simulink model "Example_UNO_Traffic_light_task"  (Simulink 3.00)
settings: Solver=ode45  SolverMode=SingleTasking  StartTime=0.0  StopTime=10.0  RelTol=1e-3
libraries: logiclib x40, mathlib x18, genlib x6, speclib x1, execlib x1
settings Model: Creator=Jarda  LastModifiedBy=XPMUser

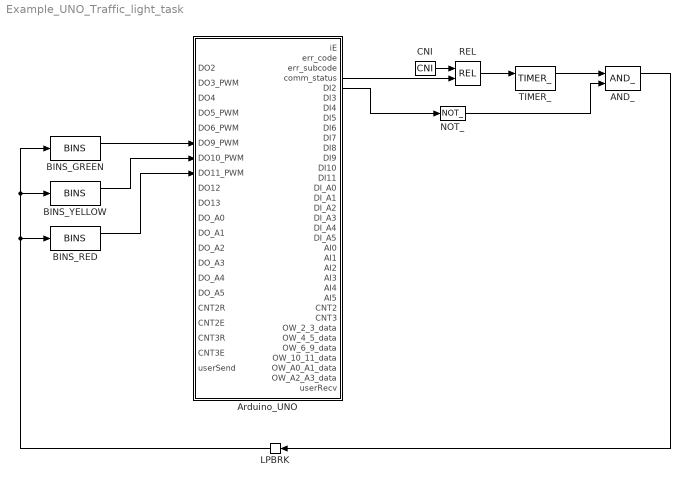
== system Example_UNO_Traffic_light_task ==
  AND_ : logiclib/AND_
  Arduino_UNO : Subsystem  mask(REX sequence){comPort=10, pinmode2=4: Digital input with internal pull-up, pinmode3=1: Not connected, pinmode4=1: Not connected, pinmode5=1: Not connected, pinmode6=1: Not connected, pinmode9=2: Digital output, pinmode10=2: Digital output, pinmode11=2: Digital output, pinmodeA0=1: Not connected, pinmodeA1=1: Not connected, pinmodeA2=1: Not connected, pinmodeA3=1: Not connected, pinmodeA4=1: Not connected, pinmodeA5=1: Not connected}
      mask prompts: comPort "COM port number"; pinmode2 "Pin 2 mode"; pinmode3 "Pin 3 mode"; pinmode4 "Pin 4 mode"; pinmode5 "Pin 5 mode"; pinmode6 "Pin 6 mode"; pinmode9 "Pin 9 mode"; pinmode10 "Pin 10 mode"; pinmode11 "Pin 11 mode"; pinmodeA0 "Analog pin A0 mode"; pinmodeA1 "Analog pin A1 mode"; pinmodeA2 "Analog pin A2 mode"; pinmodeA3 "Analog pin A3 mode"; pinmodeA4 "Analog pin A4 mode"; pinmodeA5 "Analog pin A5 mode"
      mask StyleString: popup(1|2|3|4|5|6|7|8|9|10|11|12),popup(1: Not connected|2: Digital output|3: Digital input|4: Digital input with internal pull-up|5: --- N/A for this pin ---|6: --- N/A for this pin ---|7: 1-Wire temperature|8: Counter|9: Encoder A),popup(1: Not connected|2: Digital output|3: Digital input|4: Digital input with internal pull-up|5: PWM (analog output)|6: --- N/A for this pin ---|7: 1-Wire temperature|8: Counter|9: Encoder A),popup(1: Not connected|2: Digital output|3: Digital input|4: Digital input with internal pull-up|5: --- N/A for this pin ---|6: --- N/A for this pin ---|7: 1-Wire temperature|8: --- N/A for this pin ---|9: --- N/A for this pin ---|10: Counter DIR / Encoder B),popup(1: Not connected|2: Digital output|3: Digital input|4: Digital input with internal pull-up|5: PWM (analog output)|6: --- N/A for this pin ---|7: 1-Wire temperature|8: --- N/A for this pin ---|9: --- N/A for this pin ---|10: Counter DIR / Encoder B),popup(1: Not connected|2: Digital output|3: Digital input|4: Digital input with internal pull-up|5: PWM (analog output)|6: --- N/A for this pin ---|7: 1-Wire temperature),popup(1: Not connected|2: Digital output|3: Digital input|4: Digital input with internal pull-up|5: PWM (analog output)|6: --- N/A for this pin ---|7: 1-Wire temperature),popup(1: Not connected|2: Digital output|3: Digital input|4: Digital input with internal pull-up|5: PWM (analog output)|6: --- N/A for this pin ---|7: 1-Wire temperature),popup(1: Not connected|2: Digital output|3: Digital input|4: Digital input with internal pull-up|5: PWM (analog output)|6: --- N/A for this pin ---|7: 1-Wire temperature),popup(1: Not connected|2: Digital output|3: Digital input|4: Digital input with internal pull-up|5: --- N/A for this pin ---|6: Analog input|7: 1-Wire temperature),popup(1: Not connected|2: Digital output|3: Digital input|4: Digital input with internal pull-up|5: --- N/A for this pin ---|6: Analog input|7: 1-Wire temperature),popup(1: Not connected|2: Digital output|3: Digital input|4: Digital input with internal pull-up|5: --- N/A for this pin ---|6: Analog input|7: 1-Wire temperature),popup(1: Not connected|2: Digital output|3: Digital input|4: Digital input with internal pull-up|5: --- N/A for this pin ---|6: Analog input|7: 1-Wire temperature),popup(1: Not connected|2: Digital output|3: Digital input|4: Digital input with internal pull-up|5: --- N/A for this pin ---|6: Analog input|7: 1-Wire temperature),popup(1: Not connected|2: Digital output|3: Digital input|4: Digital input with internal pull-up|5: --- N/A for this pin ---|6: Analog input|7: 1-Wire temperature)
  BINS_GREEN : genlib/BINS  Y0=on  t1=0  t2=10  t3=0  t4=4  t5=5  t6=6  t7=7  t8=8  RPT=off
  BINS_RED : genlib/BINS  Y0=off  t1=2  t2=10  t3=0  t4=4  t5=5  t6=6  t7=7  t8=8  RPT=off
  BINS_YELLOW : genlib/BINS  Y0=off  t1=0  t2=2  t3=8  t4=10  t5=0  t6=6  t7=7  t8=8  RPT=off
  CNI : mathlib/CNI  icn=3
  LPBRK : execlib/LPBRK  Orientation=left
  NOT_ : logiclib/NOT_
  REL : mathlib/REL  irel=1: equality (==)
  TIMER_ : logiclib/TIMER_  mode=2: Delayed ON  pt=1
  wires:
  AND_/1 -> LPBRK/1
  Arduino_UNO/4(comm_status) -> REL/2
  Arduino_UNO/5(DI2) -> NOT_/1
  BINS_GREEN/1 -> Arduino_UNO/6(DO9_PWM)
  BINS_RED/1 -> Arduino_UNO/8(DO11_PWM)
  BINS_YELLOW/1 -> Arduino_UNO/7(DO10_PWM)
  CNI/1 -> REL/1
  LPBRK/1 -> BINS_RED/1, BINS_GREEN/1, BINS_YELLOW/1
  NOT_/1 -> AND_/2
  REL/1 -> TIMER_/1
  TIMER_/1 -> AND_/1

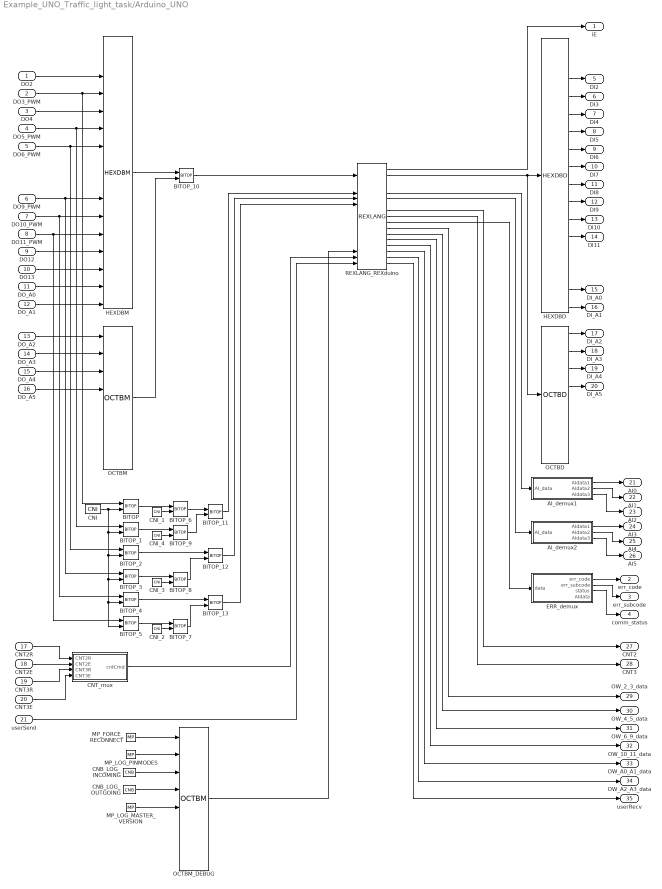
== system Example_UNO_Traffic_light_task/Arduino_UNO ==
  DO2 : Inport  Port=1
  DO3_PWM : Inport  Port=2
  DO4 : Inport  Port=3
  DO5_PWM : Inport  Port=4
  DO6_PWM : Inport  Port=5
  DO9_PWM : Inport  Port=6
  DO10_PWM : Inport  Port=7
  DO11_PWM : Inport  Port=8
  DO12 : Inport  Port=9
  DO13 : Inport  Port=10
  DO_A0 : Inport  Port=11
  DO_A1 : Inport  Port=12
  DO_A2 : Inport  Port=13
  DO_A3 : Inport  Port=14
  DO_A4 : Inport  Port=15
  DO_A5 : Inport  Port=16
  CNT2R : Inport  Port=17
  CNT2E : Inport  Port=18
  CNT3R : Inport  Port=19
  CNT3E : Inport  Port=20
  userSend : Inport  Port=21
  AI_demux1 : Subsystem
      mask Type: REX sequence
  AI_demux2 : Subsystem
      mask Type: REX sequence
  BITOP : logiclib/BITOP  SystemSampleTime=-1  iop=3: Bit AND
  BITOP_{1..5} (5 alike) : logiclib/BITOP  SystemSampleTime=-1  iop=3: Bit AND
  BITOP_{10..13} (4 alike) : logiclib/BITOP  SystemSampleTime=-1  iop=2: Bit OR
  BITOP_{6..9} (4 alike) : logiclib/BITOP  SystemSampleTime=-1  iop=5: Shift Left
  CNB_LOG_INCOMING : mathlib/CNB  SystemSampleTime=-1  YCN=off
  CNB_LOG_OUTGOING : mathlib/CNB  SystemSampleTime=-1  YCN=off
  CNI : mathlib/CNI  SystemSampleTime=-1  icn=255
  CNI_1 : mathlib/CNI  SystemSampleTime=-1  icn=8
  CNI_2 : mathlib/CNI  SystemSampleTime=-1  icn=8
  CNI_3 : mathlib/CNI  SystemSampleTime=-1  icn=24
  CNI_4 : mathlib/CNI  SystemSampleTime=-1  icn=24
  CNT_mux : Subsystem
      mask Type: REX sequence
  ERR_demux : Subsystem
      mask Type: REX sequence
  HEXDBD : logiclib/HEXDBD  SystemSampleTime=-1  shift=0
  HEXDBM : logiclib/HEXDBM  SystemSampleTime=-1  shift=0
  MP_FORCE_RECONNECT : genlib/MP  SystemSampleTime=-1  pwidth=10  BSTATE=off  RPTF=off
  MP_LOG_MASTER_VERSION : genlib/MP  SystemSampleTime=-1  pwidth=10  BSTATE=off  RPTF=off
  MP_LOG_PINMODES : genlib/MP  SystemSampleTime=-1  pwidth=10  BSTATE=off  RPTF=off
  OCTBD : logiclib/OCTBD  SystemSampleTime=-1  shift=16
  OCTBM : logiclib/OCTBM  SystemSampleTime=-1  shift=16
  OCTBM_DEBUG : logiclib/OCTBM  SystemSampleTime=-1  shift=0
  REXLANG_REXduino : speclib/REXLANG  SystemSampleTime=-1  tab_matlab=MORE  srcname=REXduino_master.stl  srctype=1: STL  stack=0  debug=1: No check  fname=REXduino_data.dat  p0=comPort  p1=pinmode2  p2=pinmode3  p3=pinmode4  p4=pinmode5  p5=pinmode6  p6=pinmode9  p7=pinmode10  p8=pinmode11  p9=pinmodeA0  p10=pinmodeA1  p11=pinmodeA2  p12=pinmodeA3  p13=pinmodeA4  p14=pinmodeA5  p15=1
  iE : Outport  Port=1
  err_code : Outport  Port=2
  err_subcode : Outport  Port=3
  comm_status : Outport  Port=4
  DI2 : Outport  Port=5
  DI3 : Outport  Port=6
  DI4 : Outport  Port=7
  DI5 : Outport  Port=8
  DI6 : Outport  Port=9
  DI7 : Outport  Port=10
  DI8 : Outport  Port=11
  DI9 : Outport  Port=12
  DI10 : Outport  Port=13
  DI11 : Outport  Port=14
  DI_A0 : Outport  Port=15
  DI_A1 : Outport  Port=16
  DI_A2 : Outport  Port=17
  DI_A3 : Outport  Port=18
  DI_A4 : Outport  Port=19
  DI_A5 : Outport  Port=20
  AI0 : Outport  Port=21
  AI1 : Outport  Port=22
  AI2 : Outport  Port=23
  AI3 : Outport  Port=24
  AI4 : Outport  Port=25
  AI5 : Outport  Port=26
  CNT2 : Outport  Port=27
  CNT3 : Outport  Port=28
  OW_2_3_data : Outport  Port=29
  OW_4_5_data : Outport  Port=30
  OW_6_9_data : Outport  Port=31
  OW_10_11_data : Outport  Port=32
  OW_A0_A1_data : Outport  Port=33
  OW_A2_A3_data : Outport  Port=34
  userRecv : Outport  Port=35
  wires:
  AI_demux1/1(AIdata1) -> AI0/1
  AI_demux1/2(AIdata2) -> AI1/1
  AI_demux1/3(AIdata3) -> AI2/1
  AI_demux2/1(AIdata1) -> AI3/1
  AI_demux2/2(AIdata2) -> AI4/1
  AI_demux2/3(AIdata3) -> AI5/1
  BITOP/1 -> BITOP_6/1
  BITOP_1/1 -> BITOP_9/1
  BITOP_10/1 -> REXLANG_REXduino/2
  BITOP_11/1 -> REXLANG_REXduino/5
  BITOP_12/1 -> REXLANG_REXduino/6
  BITOP_13/1 -> REXLANG_REXduino/7
  BITOP_2/1 -> BITOP_12/1
  BITOP_3/1 -> BITOP_8/1
  BITOP_4/1 -> BITOP_13/1
  BITOP_5/1 -> BITOP_7/1
  BITOP_6/1 -> BITOP_11/1
  BITOP_7/1 -> BITOP_13/2
  BITOP_8/1 -> BITOP_12/2
  BITOP_9/1 -> BITOP_11/2
  CNB_LOG_INCOMING/1 -> OCTBM_DEBUG/3
  CNB_LOG_OUTGOING/1 -> OCTBM_DEBUG/4
  CNI/1 -> BITOP/2, BITOP_1/2, BITOP_2/2, BITOP_3/2, BITOP_4/2, BITOP_5/2
  CNI_1/1 -> BITOP_6/2
  CNI_2/1 -> BITOP_7/2
  CNI_3/1 -> BITOP_8/2
  CNI_4/1 -> BITOP_9/2
  CNT2E/1 -> CNT_mux/2(CNT2E)
  CNT2R/1 -> CNT_mux/1(CNT2R)
  CNT3E/1 -> CNT_mux/4(CNT3E)
  CNT3R/1 -> CNT_mux/3(CNT3R)
  CNT_mux/1(cntCmd) -> REXLANG_REXduino/16
  DO10_PWM/1 -> BITOP_4/1, HEXDBM/11
  DO11_PWM/1 -> BITOP_5/1, HEXDBM/12
  DO12/1 -> HEXDBM/13
  DO13/1 -> HEXDBM/14
  DO2/1 -> HEXDBM/3
  DO3_PWM/1 -> BITOP/1, HEXDBM/4
  DO4/1 -> HEXDBM/5
  DO5_PWM/1 -> BITOP_1/1, HEXDBM/6
  DO6_PWM/1 -> BITOP_2/1, HEXDBM/7
  DO9_PWM/1 -> BITOP_3/1, HEXDBM/10
  DO_A0/1 -> HEXDBM/15
  DO_A1/1 -> HEXDBM/16
  DO_A2/1 -> OCTBM/1
  DO_A3/1 -> OCTBM/2
  DO_A4/1 -> OCTBM/3
  DO_A5/1 -> OCTBM/4
  ERR_demux/1(err_code) -> err_code/1
  ERR_demux/2(err_subcode) -> err_subcode/1
  ERR_demux/3(status) -> comm_status/1
  HEXDBD/3 -> DI2/1
  HEXDBD/4 -> DI3/1
  HEXDBD/5 -> DI4/1
  HEXDBD/6 -> DI5/1
  HEXDBD/7 -> DI6/1
  HEXDBD/8 -> DI7/1
  HEXDBD/9 -> DI8/1
  HEXDBD/10 -> DI9/1
  HEXDBD/11 -> DI10/1
  HEXDBD/12 -> DI11/1
  HEXDBD/15 -> DI_A0/1
  HEXDBD/16 -> DI_A1/1
  HEXDBM/1 -> BITOP_10/1
  MP_FORCE_RECONNECT/1 -> OCTBM_DEBUG/1
  MP_LOG_MASTER_VERSION/1 -> OCTBM_DEBUG/5
  MP_LOG_PINMODES/1 -> OCTBM_DEBUG/2
  OCTBD/1 -> DI_A2/1
  OCTBD/2 -> DI_A3/1
  OCTBD/3 -> DI_A4/1
  OCTBD/4 -> DI_A5/1
  OCTBM/1 -> BITOP_10/2
  OCTBM_DEBUG/1 -> REXLANG_REXduino/15
  REXLANG_REXduino/1 -> iE/1
  REXLANG_REXduino/2 -> HEXDBD/1, OCTBD/1
  REXLANG_REXduino/5 -> AI_demux1/1(AI_data)
  REXLANG_REXduino/6 -> AI_demux2/1(AI_data)
  REXLANG_REXduino/8 -> CNT2/1
  REXLANG_REXduino/9 -> CNT3/1
  REXLANG_REXduino/10 -> ERR_demux/1(data)
  REXLANG_REXduino/11 -> OW_2_3_data/1
  REXLANG_REXduino/12 -> OW_4_5_data/1
  REXLANG_REXduino/13 -> OW_6_9_data/1
  REXLANG_REXduino/14 -> OW_10_11_data/1
  REXLANG_REXduino/15 -> OW_A0_A1_data/1
  REXLANG_REXduino/16 -> OW_A2_A3_data/1
  REXLANG_REXduino/17 -> userRecv/1
  userSend/1 -> REXLANG_REXduino/17

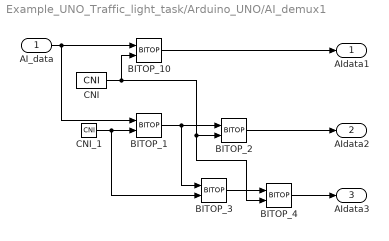
== system Example_UNO_Traffic_light_task/Arduino_UNO/AI_demux1 ==
  AI_data : Inport  Port=1
  BITOP_1 : logiclib/BITOP  SystemSampleTime=-1  iop=6: Shift Right
  BITOP_10 : logiclib/BITOP  SystemSampleTime=-1  iop=3: Bit AND
  BITOP_2 : logiclib/BITOP  SystemSampleTime=-1  iop=3: Bit AND
  BITOP_3 : logiclib/BITOP  SystemSampleTime=-1  iop=6: Shift Right
  BITOP_4 : logiclib/BITOP  SystemSampleTime=-1  iop=3: Bit AND
  CNI : mathlib/CNI  SystemSampleTime=-1  icn=1023
  CNI_1 : mathlib/CNI  SystemSampleTime=-1  icn=10
  AIdata1 : Outport  Port=1
  AIdata2 : Outport  Port=2
  AIdata3 : Outport  Port=3
  wires:
  AI_data/1 -> BITOP_1/1, BITOP_10/1
  BITOP_1/1 -> BITOP_2/1, BITOP_3/1
  BITOP_10/1 -> AIdata1/1
  BITOP_2/1 -> AIdata2/1
  BITOP_3/1 -> BITOP_4/1
  BITOP_4/1 -> AIdata3/1
  CNI/1 -> BITOP_10/2, BITOP_2/2, BITOP_4/2
  CNI_1/1 -> BITOP_1/2, BITOP_3/2

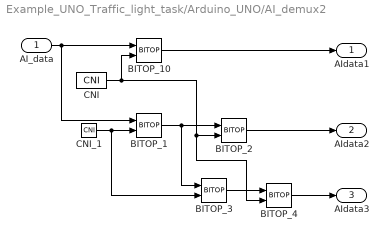
== system Example_UNO_Traffic_light_task/Arduino_UNO/AI_demux2 ==
  AI_data : Inport  Port=1
  BITOP_1 : logiclib/BITOP  SystemSampleTime=-1  iop=6: Shift Right
  BITOP_10 : logiclib/BITOP  SystemSampleTime=-1  iop=3: Bit AND
  BITOP_2 : logiclib/BITOP  SystemSampleTime=-1  iop=3: Bit AND
  BITOP_3 : logiclib/BITOP  SystemSampleTime=-1  iop=6: Shift Right
  BITOP_4 : logiclib/BITOP  SystemSampleTime=-1  iop=3: Bit AND
  CNI : mathlib/CNI  SystemSampleTime=-1  icn=1023
  CNI_1 : mathlib/CNI  SystemSampleTime=-1  icn=10
  AIdata1 : Outport  Port=1
  AIdata2 : Outport  Port=2
  AIdata3 : Outport  Port=3
  wires:
  AI_data/1 -> BITOP_1/1, BITOP_10/1
  BITOP_1/1 -> BITOP_2/1, BITOP_3/1
  BITOP_10/1 -> AIdata1/1
  BITOP_2/1 -> AIdata2/1
  BITOP_3/1 -> BITOP_4/1
  BITOP_4/1 -> AIdata3/1
  CNI/1 -> BITOP_10/2, BITOP_2/2, BITOP_4/2
  CNI_1/1 -> BITOP_1/2, BITOP_3/2

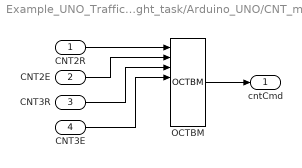
== system Example_UNO_Traffic_light_task/Arduino_UNO/CNT_mux ==
  CNT2R : Inport  Port=1
  CNT2E : Inport  Port=2
  CNT3R : Inport  Port=3
  CNT3E : Inport  Port=4
  OCTBM : logiclib/OCTBM  SystemSampleTime=-1  shift=0
  cntCmd : Outport  Port=1
  wires:
  CNT2E/1 -> OCTBM/2
  CNT2R/1 -> OCTBM/1
  CNT3E/1 -> OCTBM/4
  CNT3R/1 -> OCTBM/3
  OCTBM/1 -> cntCmd/1

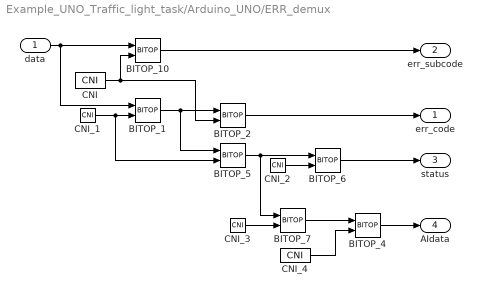
== system Example_UNO_Traffic_light_task/Arduino_UNO/ERR_demux ==
  data : Inport  Port=1
  BITOP_1 : logiclib/BITOP  SystemSampleTime=-1  iop=6: Shift Right
  BITOP_{2,4,6,10} (4 alike) : logiclib/BITOP  SystemSampleTime=-1  iop=3: Bit AND
  BITOP_5 : logiclib/BITOP  SystemSampleTime=-1  iop=6: Shift Right
  BITOP_7 : logiclib/BITOP  SystemSampleTime=-1  iop=6: Shift Right
  CNI : mathlib/CNI  SystemSampleTime=-1  icn=255
  CNI_1 : mathlib/CNI  SystemSampleTime=-1  icn=8
  CNI_2 : mathlib/CNI  SystemSampleTime=-1  icn=63
  CNI_3 : mathlib/CNI  SystemSampleTime=-1  icn=6
  CNI_4 : mathlib/CNI  SystemSampleTime=-1  icn=1023
  err_code : Outport  Port=1
  err_subcode : Outport  Port=2
  status : Outport  Port=3
  AIdata : Outport  Port=4
  wires:
  BITOP_1/1 -> BITOP_2/1, BITOP_5/1
  BITOP_10/1 -> err_subcode/1
  BITOP_2/1 -> err_code/1
  BITOP_4/1 -> AIdata/1
  BITOP_5/1 -> BITOP_6/1, BITOP_7/1
  BITOP_6/1 -> status/1
  BITOP_7/1 -> BITOP_4/1
  CNI/1 -> BITOP_10/2, BITOP_2/2
  CNI_1/1 -> BITOP_1/2, BITOP_5/2
  CNI_2/1 -> BITOP_6/2
  CNI_3/1 -> BITOP_7/2
  CNI_4/1 -> BITOP_4/2
  data/1 -> BITOP_1/1, BITOP_10/1
